simulink model "p5_linearWindTurbineModel"  (R2019b)
settings: Solver=ode4  StartTime=0.0  StopTime=TIME_SIM  FixedStep=STEP_SIZE  RelTol=1e-3
values from neighbouring files (symbols this model uses):
  Ts = 0.05    [relevantWindTurbineParameters.mat]
undefined symbols (not defined in the file or in its folder): Aa, Bb, Bv, CcO, Dd, Ff, Gg, L
settings Model: Creator=Aleks  LastModifiedBy=MSI
settings DataIOCC: ReturnWorkspaceOutputs=off
settings DebuggingCC: ArithmeticOperatorsInVariantConditions=warning
settings SFSimCC: SimUseLocalCustomCode=off  CustomCodeUndefinedFunction=UseInterfaceOnly
settings RTWCC: RTWUseLocalCustomCode=off
settings CodeAppCC: StateflowObjectComments=on

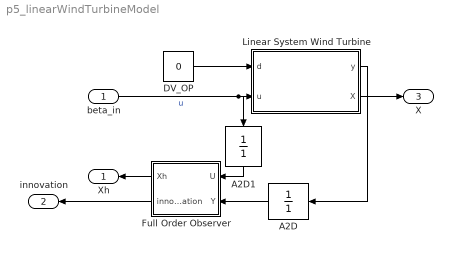
== system p5_linearWindTurbineModel ==
  beta_in : Inport
  A2D : DiscreteTransferFcn  Denominator=[1]  SampleTime=Ts
  A2D1 : DiscreteTransferFcn  Denominator=[1]  SampleTime=Ts
  DV_OP : Constant  Value=0
  Full Order Observer : Subsystem
  Linear System Wind Turbine : Subsystem
  Xh : Outport
  innovation : Outport  Port=2
  X : Outport  Port=3
  wires:
  Linear System Wind Turbine/1(y) -> A2D/1
  DV_OP/1 -> Linear System Wind Turbine/1(d)
  beta_in/1 -> Linear System Wind Turbine/2(u), A2D1/1  "u"
  Full Order Observer/1(Xh) -> Xh/1
  Full Order Observer/2(innovation) -> innovation/1
  A2D/1 -> Full Order Observer/2(Y)
  A2D1/1 -> Full Order Observer/1(U)
  Linear System Wind Turbine/2(X) -> X/1

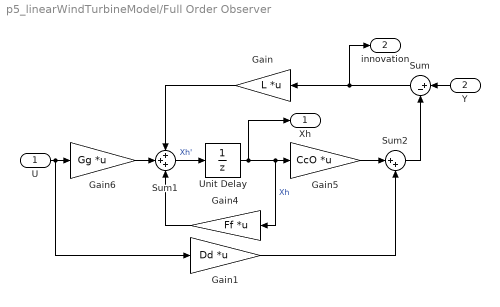
== system p5_linearWindTurbineModel/Full Order Observer ==
  U : Inport
  Y : Inport  Port=2
  Gain : Gain  Gain=L  Multiplication=Matrix(K*u) (u vector)
  Gain1 : Gain  Gain=Dd  Multiplication=Matrix(K*u) (u vector)
  Gain4 : Gain  Gain=Ff  Multiplication=Matrix(K*u) (u vector)
  Gain5 : Gain  Gain=CcO  Multiplication=Matrix(K*u) (u vector)
  Gain6 : Gain  Gain=Gg  Multiplication=Matrix(K*u) (u vector)
  Sum : Sum  Inputs=|+-
  Sum1 : Sum  Inputs=+++
  Sum2 : Sum  Inputs=|++
  Unit Delay : UnitDelay  SampleTime=Ts  HasFrameUpgradeWarning=on
  Xh : Outport
  innovation : Outport  Port=2
  wires:
  Gain4/1 -> Sum1/3
  Gain6/1 -> Sum1/2
  Sum1/1 -> Unit Delay/1  "Xh'"
  Unit Delay/1 -> Xh/1, Gain4/1, Gain5/1  "Xh"
  U/1 -> Gain1/1, Gain6/1
  Gain/1 -> Sum1/1
  Y/1 -> Sum/1
  Sum/1 -> innovation/1, Gain/1
  Gain1/1 -> Sum2/2
  Gain5/1 -> Sum2/1
  Sum2/1 -> Sum/2

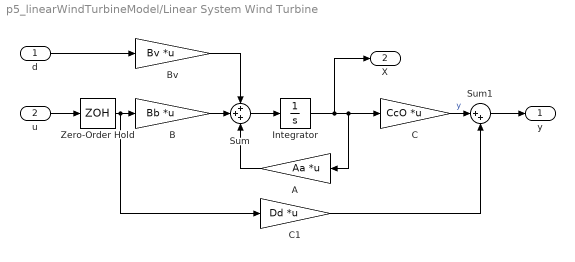
== system p5_linearWindTurbineModel/Linear System Wind Turbine ==
  d : Inport
  u : Inport  Port=2
  A : Gain  Gain=Aa  Multiplication=Matrix(K*u) (u vector)
  B : Gain  Gain=Bb  Multiplication=Matrix(K*u) (u vector)
  Bv : Gain  Gain=Bv  Multiplication=Matrix(K*u) (u vector)
  C : Gain  Gain=CcO  Multiplication=Matrix(K*u) (u vector)
  C1 : Gain  Gain=Dd  Multiplication=Matrix(K*u) (u vector)
  Integrator : Integrator
  Sum : Sum  Inputs=+++
  Sum1 : Sum  Inputs=|++
  Zero-Order Hold : ZeroOrderHold  SampleTime=Ts
  y : Outport
  X : Outport  Port=2
  wires:
  Bv/1 -> Sum/1
  Sum/1 -> Integrator/1
  Integrator/1 -> X/1, A/1, C/1
  u/1 -> Zero-Order Hold/1
  A/1 -> Sum/3
  Zero-Order Hold/1 -> C1/1, B/1
  B/1 -> Sum/2
  C/1 -> Sum1/1  "y"
  d/1 -> Bv/1
  C1/1 -> Sum1/2
  Sum1/1 -> y/1
